simulink model "ADMIRE"  (R2021b)
settings: Solver=ode4  StartTime=0.0  StopTime=100  FixedStep=1e-2  RelTol=1e-3
undefined symbols (not defined in the file or in its folder): admireDB, Earth, WGS84
libraries: simulink_extras x112, simulink x27, aerolibutil x4, dspsigops x4, aerolibfltsims x3, sharedtransform x2, aerolibtransform2 x2, aerolibatmos2 x1, matrix_library x1, sharedutil x1, aerolibanimutils x1, vrlib x1
(part 2 of 15)

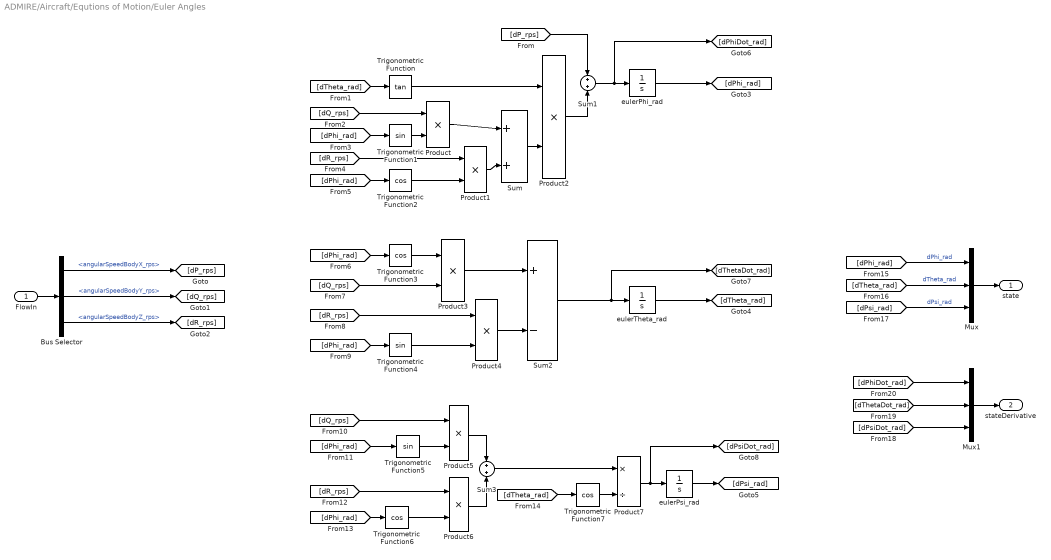
== system ADMIRE/Aircraft/Equtions of Motion/Euler Angles ==
  FlowIn : Inport
  Bus Selector : BusSelector  OutputSignals=EOM_Bus.angularSpeedBodyX_rps,EOM_Bus.angularSpeedBodyY_rps,EOM_Bus.angularSpeedBodyZ_rps
  Mux : Mux  Inputs=3
  Mux1 : Mux  Inputs=3
  Product{,1..6} (7 alike) : Product
  Product7 : Product  Inputs=*/
  Sum : Sum  Inputs=+|+
  Sum1 : Sum  Inputs=+|+
  Sum2 : Sum  Inputs=+-
  Sum3 : Sum  Inputs=+|+
  Trigonometric Function : Trigonometry  Operator=tan
  Trigonometric Function1 : Trigonometry
  Trigonometric Function{2..3,6..7} (4 alike) : Trigonometry  Operator=cos
  Trigonometric Function4 : Trigonometry
  Trigonometric Function5 : Trigonometry
  eulerPhi_rad : Integrator  WrapState=on  ContinuousStateAttributes='eulerPhi_rad'
  eulerPsi_rad : Integrator  WrapState=on  WrappedStateUpperValue=2*pi  WrappedStateLowerValue=0  ContinuousStateAttributes='eulerPsi_rad'
  eulerTheta_rad : Integrator  WrapState=on  WrappedStateUpperValue=pi/2  WrappedStateLowerValue=-pi/2  ContinuousStateAttributes='eulerTheta_rad'
  state : Outport
  stateDerivative : Outport  Port=2
  wires:
  Mux/1 -> state/1
  [dR_rps] -> Product1/1
  eulerPhi_rad/1 -> [dPhi_rad]
  [dTheta_rad] -> Mux/2  "dTheta_rad"
  Trigonometric Function7/1 -> Product7/2
  Sum1/1 -> [dPhiDot_rad], eulerPhi_rad/1
  [dPsi_rad] -> Mux/3  "dPsi_rad"
  [dPhi_rad] -> Mux/1  "dPhi_rad"
  Product4/1 -> Sum2/2
  Product6/1 -> Sum3/2
  Sum2/1 -> [dThetaDot_rad], eulerTheta_rad/1
  [dPhi_rad] -> Trigonometric Function1/1
  Product5/1 -> Sum3/1
  Trigonometric Function4/1 -> Product4/2
  [dPhi_rad] -> Trigonometric Function2/1
  Trigonometric Function6/1 -> Product6/2
  Product3/1 -> Sum2/1
  [dQ_rps] -> Product3/2
  [dPhi_rad] -> Trigonometric Function6/1
  Trigonometric Function5/1 -> Product5/2
  [dPhi_rad] -> Trigonometric Function5/1
  Product1/1 -> Sum/2
  [dR_rps] -> Product4/1
  Trigonometric Function2/1 -> Product1/2
  [dTheta_rad] -> Trigonometric Function/1
  Sum/1 -> Product2/2
  Trigonometric Function1/1 -> Product/2
  Trigonometric Function/1 -> Product2/1
  Product2/1 -> Sum1/2
  eulerTheta_rad/1 -> [dTheta_rad]
  Sum3/1 -> Product7/1
  [dTheta_rad] -> Trigonometric Function7/1
  [dQ_rps] -> Product/1
  [dR_rps] -> Product6/1
  [dP_rps] -> Sum1/1
  Product/1 -> Sum/1
  [dPhi_rad] -> Trigonometric Function3/1
  [dPhi_rad] -> Trigonometric Function4/1
  Product7/1 -> eulerPsi_rad/1, [dPsiDot_rad]
  Trigonometric Function3/1 -> Product3/1
  eulerPsi_rad/1 -> [dPsi_rad]
  [dQ_rps] -> Product5/1
  FlowIn/1 -> Bus Selector/1
  Bus Selector/3 -> [dR_rps]  "<angularSpeedBodyZ_rps>"
  Bus Selector/2 -> [dQ_rps]  "<angularSpeedBodyY_rps>"
  Bus Selector/1 -> [dP_rps]  "<angularSpeedBodyX_rps>"
  [dPhiDot_rad] -> Mux1/1
  [dThetaDot_rad] -> Mux1/2
  [dPsiDot_rad] -> Mux1/3
  Mux1/1 -> stateDerivative/1

== system ADMIRE/Aircraft/Equtions of Motion/Navigation ==
  FlowIn : Inport
  Bus Selector : BusSelector  OutputSignals=DCM_Bus.dcmBody2NED,EOM_Bus.speedBodyX_mps,EOM_Bus.speedBodyY_mps,EOM_Bus.speedBodyZ_mps
  Demux : Demux  Outputs=3
  Gain : Gain  Gain=-1
  Matrix Multiply : Product  Multiplication=Matrix(*)
  Mux : Mux  Inputs=3
  Mux1 : Mux  Inputs=3
  altitude_m : Integrator  ContinuousStateAttributes='altitude_m'
  positionEarthX_m : Integrator  ContinuousStateAttributes='positionEarthX_m'
  positionEarthY_m : Integrator  ContinuousStateAttributes='positionEarthY_m'
  state : Outport
  stateDerivative : Outport  Port=2
  wires:
  FlowIn/1 -> Bus Selector/1
  Bus Selector/2 -> Mux/1  "<speedBodyX_mps>"
  Bus Selector/3 -> Mux/2  "<speedBodyY_mps>"
  Bus Selector/4 -> Mux/3  "<speedBodyZ_mps>"
  Bus Selector/1 -> Matrix Multiply/1  "<dcmBody2NED>"
  Mux/1 -> Matrix Multiply/2
  Matrix Multiply/1 -> stateDerivative/1, Demux/1
  Demux/1 -> positionEarthX_m/1
  Demux/2 -> positionEarthY_m/1
  Demux/3 -> Gain/1
  positionEarthY_m/1 -> Mux1/2
  positionEarthX_m/1 -> Mux1/1
  altitude_m/1 -> Mux1/3
  Mux1/1 -> state/1
  Gain/1 -> altitude_m/1

== system ADMIRE/Aircraft/Equtions of Motion/Translational Speeds ==
  Flow : Inport
  Angle of Attack Equation : Subsystem
  Angle of Sideslip Equation : Subsystem
  ForcesWindAxes : Subsystem
  Mux : Mux  Inputs=6
  Selector : Selector  InputPortWidth=6  IndexOptions=Index vector (dialog)  Indices=[1 3 5]  OutputSizes=1
  Selector1 : Selector  InputPortWidth=6  IndexOptions=Index vector (dialog)  Indices=[2 4 6]  OutputSizes=1
  V Equation : Subsystem
  state : Outport
  stateDerivative : Outport  Port=2
  wires:
  V Equation/1(V) -> Mux/1  "V"
  Angle of Sideslip Equation/1(aos) -> Mux/5  "aos"
  Angle of Attack Equation/1(aoa) -> Mux/3  "aoa"
  Flow/1 -> Angle of Sideslip Equation/2(Flow), Angle of Attack Equation/2(Flow), V Equation/2(Flow), ForcesWindAxes/1(Flow)
  Mux/1 -> Selector1/1, Selector/1
  V Equation/2(VDot) -> Mux/2  "VDot"
  Angle of Attack Equation/2(aoaDot) -> Mux/4  "aoaDot"
  Angle of Sideslip Equation/2(aosDot) -> Mux/6  "aosDot"
  Selector/1 -> state/1
  Selector1/1 -> stateDerivative/1
  ForcesWindAxes/1(ForcesWindAxes) -> Angle of Attack Equation/1(ForcesWindAxes), Angle of Sideslip Equation/1(ForcesWindAxes), V Equation/1(ForcesWindAxes)

== system ADMIRE/Aircraft/Mass/Inertia ==
  Create 3x3 Matrix : sharedutil/Create 3x3 Matrix  aMode=aMode
      settings: SourceProductBaseCode=AE,PW,DR,MT,UV,VE
  Gain : Gain  Gain=-1
  Gain1 : Gain  Gain=-1
  Gain2 : Gain  Gain=-1
  "Ix " : Constant  Value=21000
  Ixy : Constant  Value=0
  "Ixz " : Constant  Value=2500
  "Iy " : Constant  Value=81000
  Iyz : Constant  Value=0
  "Iz " : Constant  Value=101000
  InertiaTensor : Outport
  inertiaIx_kgpm2 : Outport  Port=2
  inertiaIy_kgpm2 : Outport  Port=3
  inertiaIz_kgpm2 : Outport  Port=4
  inertiaIxy_kgpm2 : Outport  Port=5
  inertiaIxz_kgpm2 : Outport  Port=6
  inertiaIyz_kgpm2 : Outport  Port=7
  wires:
  "Ix "/1 -> Create 3x3 Matrix/1, [Ix]
  "Iz "/1 -> [Iz], Create 3x3 Matrix/9
  Gain2/1 -> Create 3x3 Matrix/6, Create 3x3 Matrix/8
  [Iy] -> inertiaIy_kgpm2/1  "inertiaIy_kgpm2"
  "Ixz "/1 -> [Ixz], Gain1/1
  Ixy/1 -> [Ixy], Gain/1
  Create 3x3 Matrix/1 -> InertiaTensor/1  "InertiaTensor"
  [Ix] -> inertiaIx_kgpm2/1  "inertiaIx_kgpm2"
  Gain/1 -> Create 3x3 Matrix/4, Create 3x3 Matrix/2
  [Iyz] -> inertiaIyz_kgpm2/1  "inertiaIyz_kgpm2"
  Gain1/1 -> Create 3x3 Matrix/7, Create 3x3 Matrix/3
  "Iy "/1 -> [Iy], Create 3x3 Matrix/5
  Iyz/1 -> [Iyz], Gain2/1
  [Ixz] -> inertiaIxz_kgpm2/1  "inertiaIxz_kgpm2"
  [Ixy] -> inertiaIxy_kgpm2/1  "inertiaIxy_kgpm2"
  [Iz] -> inertiaIz_kgpm2/1  "inertiaIz_kgpm2"

== system ADMIRE/InputSelection/LogitechExtremePro3D/Subsystem ==
  JoyInput : Inport
  TrimInput : Inport  Port=2
  Constant1 : Constant
  Gain : Gain  Gain=20
  Integrator : Integrator  InitialConditionSource=external
  Sample and Hold : dspsigops/Sample and Hold  trig=Either edge  initCond=0  latchinput=off
  Sum : Sum  Inputs=|+-
  Switch : Switch  Criteria=u2 > Threshold
  Out : Outport
  wires:
  Constant1/1 -> Sample and Hold/1
  Sample and Hold/1 -> Switch/2
  JoyInput/1 -> Sample and Hold/Trigger, Switch/1
  Switch/1 -> Sum/1
  TrimInput/1 -> Integrator/2, Switch/3
  Integrator/1 -> Out/1, Sum/2
  Sum/1 -> Gain/1
  Gain/1 -> Integrator/1

== system ADMIRE/InputSelection/LogitechExtremePro3D/Subsystem1 ==
  JoyInput : Inport
  TrimInput : Inport  Port=2
  Constant1 : Constant
  Gain : Gain  Gain=20
  Integrator : Integrator  InitialConditionSource=external
  Sample and Hold : dspsigops/Sample and Hold  trig=Either edge  initCond=0  latchinput=off
  Sum : Sum  Inputs=|+-
  Switch : Switch  Criteria=u2 > Threshold
  Out : Outport
  wires:
  Gain/1 -> Integrator/1
  Sum/1 -> Gain/1
  Integrator/1 -> Sum/2, Out/1
  TrimInput/1 -> Switch/3, Integrator/2
  Switch/1 -> Sum/1
  JoyInput/1 -> Switch/1, Sample and Hold/Trigger
  Sample and Hold/1 -> Switch/2
  Constant1/1 -> Sample and Hold/1

== system ADMIRE/InputSelection/LogitechExtremePro3D/Subsystem2 ==
  JoyInput : Inport
  TrimInput : Inport  Port=2
  Constant1 : Constant
  Gain : Gain  Gain=20
  Integrator : Integrator  InitialConditionSource=external
  Sample and Hold : dspsigops/Sample and Hold  trig=Either edge  initCond=0  latchinput=off
  Sum : Sum  Inputs=|+-
  Switch : Switch  Criteria=u2 > Threshold
  Out : Outport
  wires:
  Constant1/1 -> Sample and Hold/1
  Sample and Hold/1 -> Switch/2
  JoyInput/1 -> Sample and Hold/Trigger, Switch/1
  Switch/1 -> Sum/1
  TrimInput/1 -> Integrator/2, Switch/3
  Integrator/1 -> Out/1, Sum/2
  Sum/1 -> Gain/1
  Gain/1 -> Integrator/1

== system ADMIRE/InputSelection/LogitechExtremePro3D/Subsystem3 ==
  JoyInput : Inport
  TrimInput : Inport  Port=2
  Constant1 : Constant
  Gain : Gain  Gain=20
  Integrator : Integrator  InitialConditionSource=external
  Sample and Hold : dspsigops/Sample and Hold  trig=Either edge  initCond=0  latchinput=off
  Sum : Sum  Inputs=|+-
  Switch : Switch  Criteria=u2 > Threshold
  Out : Outport
  wires:
  Gain/1 -> Integrator/1
  Sum/1 -> Gain/1
  Integrator/1 -> Sum/2, Out/1
  TrimInput/1 -> Switch/3, Integrator/2
  Switch/1 -> Sum/1
  JoyInput/1 -> Switch/1, Sample and Hold/Trigger
  Sample and Hold/1 -> Switch/2
  Constant1/1 -> Sample and Hold/1

== system ADMIRE/Aircraft/Aerodynamics/CentripetalForceCoefficient/MachRegion1 ==
  note: Mach <= 0.4
  AeroIn_Bus : Inport
  Bus Creator : BusCreator  Inputs=3
  Ccbcai : Subsystem
  Ccbde : Subsystem
  Ccbdle : Subsystem
  Ccbdn : Subsystem
  Ccbeta : Subsystem
  Ccbetad : Subsystem
  Ccblg : Subsystem
  Ccdai : Subsystem
  Ccdaib : Subsystem
  Ccday : Subsystem
  Ccdayb : Subsystem
  Ccdna : Subsystem
  Ccdr : Subsystem
  Ccp : Subsystem
  Ccpbeta : Subsystem
  Ccr : Subsystem
  Ccrbeta : Subsystem
  Sum : Sum  Inputs=17
  eoeff1 : Subsystem
  cctot : Outport
  wires:
  Ccrbeta/1(Ccrbeta) -> Sum/17  "Ccrbeta"
  Ccr/1(Ccr) -> Sum/16  "Ccr"
  Ccpbeta/1(Ccpbeta) -> Sum/15  "Ccpbeta"
  Ccp/1(Ccp) -> Sum/14  "Ccp"
  Ccbetad/1(Ccbetad) -> Sum/13  "Ccbetad"
  Ccdna/1(Ccdna) -> Sum/12  "Ccdna"
  Ccdayb/1(Ccdayb) -> Sum/11  "Ccdayb"
  Ccday/1(Ccday) -> Sum/10  "Ccday"
  Ccdaib/1(Ccdaib) -> Sum/9  "Ccdaib"
  Ccdai/1(Ccdai) -> Sum/8  "Ccdai"
  Ccdr/1(Ccdr) -> Sum/7  "Ccdr"
  Ccbcai/1(Ccbcai) -> Sum/6  "Ccbcai"
  Ccbdle/1(Ccbdle) -> Sum/5  "Ccbdle"
  Ccbdn/1(Ccbdn) -> Sum/4  "Ccbdn"
  Ccbde/1(Ccbde) -> Sum/3  "Ccbde"
  Ccblg/1(Ccblg) -> Sum/2  "Ccblg"
  Ccbeta/1(Ccbeta) -> Sum/1  "Ccbeta"
  Bus Creator/1 -> Ccp/1(in_bus), Ccpbeta/1(in_bus), Ccr/1(in_bus), Ccrbeta/1(in_bus), Ccbetad/1(in_bus), Ccdna/1(in_bus), Ccdayb/1(in_bus), Ccday/1(in_bus), Ccdaib/1(in_bus), Ccdai/1(in_bus), Ccdr/1(in_bus), Ccbcai/1(in_bus), Ccbdle/1(in_bus), Ccbdn/1(in_bus), Ccbde/1(in_bus), Ccblg/1(in_bus), Ccbeta/1(in_bus)  "in_bus"
  eoeff1/2(eieff) -> Bus Creator/3  "eieff"
  AeroIn_Bus/1 -> eoeff1/1(AeroIn_Bus), Bus Creator/1
  eoeff1/1(eoeff) -> Bus Creator/2  "eoeff"
  Sum/1 -> cctot/1

== system ADMIRE/Aircraft/Aerodynamics/CentripetalForceCoefficient/MachRegion2 ==
  note: 0.4 < Mach < 0.5
  AeroIn_Bus : Inport
  Bus Creator : BusCreator  Inputs=3
  Ccbcai : Subsystem
  Ccbde : Subsystem
  Ccbdle : Subsystem
  Ccbdn : Subsystem
  Ccbeta : Subsystem
  Ccbetad : Subsystem
  Ccblg : Subsystem
  Ccdai : Subsystem
  Ccdaib : Subsystem
  Ccday : Subsystem
  Ccdayb : Subsystem
  Ccdna : Subsystem
  Ccdr : Subsystem
  Ccp : Subsystem
  Ccpbeta : Subsystem
  Ccr : Subsystem
  Ccrbeta : Subsystem
  Sum : Sum  Inputs=17
  eoeff1 : Subsystem
  cctot : Outport
  wires:
  Ccrbeta/1(Ccrbeta) -> Sum/17  "Ccrbeta"
  Ccr/1(Ccr) -> Sum/16  "Ccr"
  Ccpbeta/1(Ccpbeta) -> Sum/15  "Ccpbeta"
  Ccp/1(Ccp) -> Sum/14  "Ccp"
  Ccbetad/1(Ccbetad) -> Sum/13  "Ccbetad"
  Ccdna/1(Ccdna) -> Sum/12  "Ccdna"
  Ccdayb/1(Ccdayb) -> Sum/11  "Ccdayb"
  Ccday/1(Ccday) -> Sum/10  "Ccday"
  Ccdaib/1(Ccdaib) -> Sum/9  "Ccdaib"
  Ccdai/1(Ccdai) -> Sum/8  "Ccdai"
  Ccdr/1(Ccdr) -> Sum/7  "Ccdr"
  Ccbcai/1(Ccbcai) -> Sum/6  "Ccbcai"
  Ccbdle/1(Ccbdle) -> Sum/5  "Ccbdle"
  Ccbdn/1(Ccbdn) -> Sum/4  "Ccbdn"
  Ccbde/1(Ccbde) -> Sum/3  "Ccbde"
  Ccblg/1(Ccblg) -> Sum/2  "Ccblg"
  Ccbeta/1(Ccbeta) -> Sum/1  "Ccbeta"
  Bus Creator/1 -> Ccr/1(in_bus), Ccrbeta/1(in_bus), Ccpbeta/1(in_bus), Ccp/1(in_bus), Ccbetad/1(in_bus), Ccdna/1(in_bus), Ccdayb/1(in_bus), Ccday/1(in_bus), Ccdaib/1(in_bus), Ccdai/1(in_bus), Ccdr/1(in_bus), Ccbcai/1(in_bus), Ccbdle/1(in_bus), Ccbdn/1(in_bus), Ccbde/1(in_bus), Ccblg/1(in_bus), Ccbeta/1(in_bus)  "in_bus"
  eoeff1/1(eoeff) -> Bus Creator/2  "eoeff"
  eoeff1/2(eieff) -> Bus Creator/3  "eieff"
  AeroIn_Bus/1 -> eoeff1/1(AeroIn_Bus), Bus Creator/1
  Sum/1 -> cctot/1

== system ADMIRE/Aircraft/Aerodynamics/CentripetalForceCoefficient/MachRegion3 ==
  note: 0.5 <= Mach <= 1.4
  AeroIn_Bus : Inport
  Bus Creator : BusCreator  Inputs=3
  Ccbcai : Subsystem
  Ccbde : Subsystem
  Ccbdle : Subsystem
  Ccbdn : Subsystem
  Ccbeta : Subsystem
  Ccbetad : Subsystem
  Ccblg : Subsystem
  Ccdai : Subsystem
  Ccdaib : Subsystem
  Ccday : Subsystem
  Ccdayb : Subsystem
  Ccdna : Subsystem
  Ccdr : Subsystem
  Ccp1 : Subsystem
  Ccpbeta : Subsystem
  Ccr1 : Subsystem
  Ccrbeta : Subsystem
  Sum : Sum  Inputs=17
  eoeff1 : Subsystem
  cctot : Outport
  wires:
  Ccrbeta/1(Ccrbeta) -> Sum/17  "Ccrbeta"
  Ccr1/1(Ccr) -> Sum/16  "Ccr"
  Ccpbeta/1(Ccpbeta) -> Sum/15  "Ccpbeta"
  Ccp1/1(Ccp) -> Sum/14  "Ccp"
  Ccbetad/1(Ccbetad) -> Sum/13  "Ccbetad"
  Ccdna/1(Ccdna) -> Sum/12  "Ccdna"
  Ccdayb/1(Ccdayb) -> Sum/11  "Ccdayb"
  Ccday/1(Ccday) -> Sum/10  "Ccday"
  Ccdaib/1(Ccdaib) -> Sum/9  "Ccdaib"
  Ccdai/1(Ccdai) -> Sum/8  "Ccdai"
  Ccdr/1(Ccdr) -> Sum/7  "Ccdr"
  Ccbcai/1(Ccbcai) -> Sum/6  "Ccbcai"
  Ccbdle/1(Ccbdle) -> Sum/5  "Ccbdle"
  Ccbdn/1(Ccbdn) -> Sum/4  "Ccbdn"
  Ccbde/1(Ccbde) -> Sum/3  "Ccbde"
  Ccblg/1(Ccblg) -> Sum/2  "Ccblg"
  Ccbeta/1(Ccbeta) -> Sum/1  "Ccbeta"
  eoeff1/2(eieff) -> Bus Creator/3  "eieff"
  eoeff1/1(eoeff) -> Bus Creator/2  "eoeff"
  Bus Creator/1 -> Ccr1/1(in_bus), Ccp1/1(in_bus), Ccbetad/1(in_bus), Ccdna/1(in_bus), Ccday/1(in_bus), Ccdai/1(in_bus), Ccdr/1(in_bus), Ccbcai/1(in_bus), Ccbdle/1(in_bus), Ccbdn/1(in_bus), Ccbde/1(in_bus), Ccblg/1(in_bus), Ccbeta/1(in_bus)  "in_bus"
  AeroIn_Bus/1 -> eoeff1/1(AeroIn_Bus), Bus Creator/1
  Sum/1 -> cctot/1

== system ADMIRE/Aircraft/Aerodynamics/CentripetalForceCoefficient/MachRegion4 ==
  note: 1.4 < Mach
  AeroIn_Bus : Inport
  Bus Creator : BusCreator  Inputs=3
  Ccbcai : Subsystem
  Ccbde : Subsystem
  Ccbdle : Subsystem
  Ccbdn : Subsystem
  Ccbeta : Subsystem
  Ccbetad : Subsystem
  Ccblg : Subsystem
  Ccdai : Subsystem
  Ccdaib : Subsystem
  Ccday : Subsystem
  Ccdayb : Subsystem
  Ccdna : Subsystem
  Ccdr : Subsystem
  Ccp : Subsystem
  Ccpbeta : Subsystem
  Ccr : Subsystem
  Ccrbeta : Subsystem
  Sum : Sum  Inputs=17
  eoeff : Subsystem
  cttot : Outport
  wires:
  Ccrbeta/1(Ccrbeta) -> Sum/17  "Ccrbeta"
  Ccr/1(Ccr) -> Sum/16  "Ccr"
  Ccpbeta/1(Ccpbeta) -> Sum/15  "Ccpbeta"
  Ccp/1(Ccp) -> Sum/14  "Ccp"
  Ccbetad/1(Ccbetad) -> Sum/13  "Ccbetad"
  Ccdna/1(Ccdna) -> Sum/12  "Ccdna"
  Ccdayb/1(Ccdayb) -> Sum/11  "Ccdayb"
  Ccday/1(Ccday) -> Sum/10  "Ccday"
  Ccdaib/1(Ccdaib) -> Sum/9  "Ccdaib"
  Ccdai/1(Ccdai) -> Sum/8  "Ccdai"
  Ccblg/1(Ccblg) -> Sum/7  "Ccblg"
  Ccdr/1(Ccdr) -> Sum/6  "Ccdr"
  Ccbcai/1(Ccbcai) -> Sum/5  "Ccbcai"
  Ccbdle/1(Ccbdle) -> Sum/4  "Ccbdle"
  Ccbdn/1(Ccbdn) -> Sum/3  "Ccbdn"
  Ccbde/1(Ccbde) -> Sum/2  "Ccbde"
  Ccbeta/1(Ccbeta) -> Sum/1  "Ccbeta"
  AeroIn_Bus/1 -> eoeff/1(AeroIn_Bus), Bus Creator/1
  Bus Creator/1 -> Ccbde/1(in_bus), Ccbdn/1(in_bus), Ccbdle/1(in_bus), Ccbcai/1(in_bus), Ccdr/1(in_bus), Ccr/1(in_bus), Ccp/1(in_bus), Ccbetad/1(in_bus), Ccdna/1(in_bus), Ccday/1(in_bus), Ccdai/1(in_bus), Ccblg/1(in_bus), Ccbeta/1(in_bus)  "in_bus"
  eoeff/2(eieff) -> Bus Creator/3  "eieff"
  eoeff/1(eoeff) -> Bus Creator/2  "eoeff"
  Sum/1 -> cttot/1

== system ADMIRE/Aircraft/Aerodynamics/CentripetalForceCoefficient/Subsystem ==
  mach_nd : Inport
  CctotMR1 : Inport  Port=2
  CctotMR2 : Inport  Port=3
  CctotMR3 : Inport  Port=4
  CctotMR4 : Inport  Port=5
  AND : Logic  IconShape=distinctive  AllPortsSameDT=off  OutDataTypeStr=boolean
  AND1 : Logic  IconShape=distinctive  AllPortsSameDT=off  OutDataTypeStr=boolean
  Compare To Constant1 : simulink/Logic and Bit Operations/Compare To Constant  relop=<=  const=0.4  OutDataTypeStr=boolean
  Compare To Constant2 : simulink/Logic and Bit Operations/Compare To Constant  relop=>  const=0.4  OutDataTypeStr=boolean
  Compare To Constant3 : simulink/Logic and Bit Operations/Compare To Constant  relop=<  const=0.5  OutDataTypeStr=boolean
  Compare To Constant4 : simulink/Logic and Bit Operations/Compare To Constant  relop=<=  const=1.4  OutDataTypeStr=boolean
  Compare To Constant5 : simulink/Logic and Bit Operations/Compare To Constant  relop=>=  const=0.5  OutDataTypeStr=boolean
  Switch : Switch  Criteria=u2 ~= 0
  Switch1 : Switch  Criteria=u2 ~= 0
  Switch2 : Switch  Criteria=u2 ~= 0
  Cctot : Outport
  wires:
  Switch/1 -> Cctot/1
  Compare To Constant5/1 -> AND1/1
  Compare To Constant4/1 -> AND1/2
  AND1/1 -> Switch2/2
  CctotMR4/1 -> Switch2/3
  CctotMR3/1 -> Switch2/1
  CctotMR1/1 -> Switch/1
  Switch2/1 -> Switch1/3
  CctotMR2/1 -> Switch1/1
  Switch1/1 -> Switch/3
  AND/1 -> Switch1/2
  Compare To Constant3/1 -> AND/2
  Compare To Constant2/1 -> AND/1
  Compare To Constant1/1 -> Switch/2
  mach_nd/1 -> Compare To Constant1/1, Compare To Constant3/1, Compare To Constant4/1, Compare To Constant5/1, Compare To Constant2/1

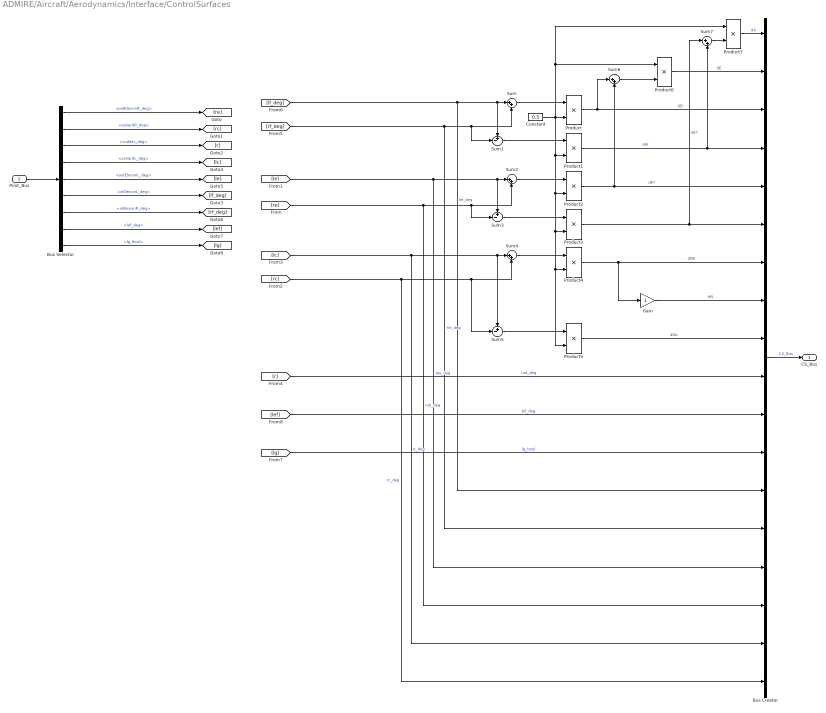
== system ADMIRE/Aircraft/Aerodynamics/Interface/ControlSurfaces ==
  Pilot_Bus : Inport
  Bus Creator : BusCreator  Inputs=18
  Bus Selector : BusSelector  OutputSignals=CS_Bus.outElevonR_deg,CS_Bus.canardR_deg,CS_Bus.rudder_deg,CS_Bus.canardL_deg,CS_Bus.outElevonL_deg,CS_Bus.inElevonL_deg,CS_Bus.inElevonR_deg,CS_Bus.lef_deg,CS_Bus.lg_bool
  Constant : Constant  Value=0.5
  Gain : Gain
  Product{,1..7} (8 alike) : Product
  Sum{,2,4,6..7} (5 alike) : Sum  Inputs=|++
  Sum1 : Sum  Inputs=+-|
  Sum3 : Sum  Inputs=+-|
  Sum5 : Sum  Inputs=+-|
  CS_Bus : Outport
  wires:
  Product/1 -> Sum6/1, Bus Creator/3  "dEI"
  [lf_deg] -> Bus Creator/13, Sum1/1, Sum/1  "lie_deg"
  Product1/1 -> Sum7/2, Bus Creator/4  "dAI"
  Product2/1 -> Sum6/2, Bus Creator/5  "dEY"
  Product3/1 -> Bus Creator/6, Sum7/1  "dAY"
  Product5/1 -> Bus Creator/9  "dNA"
  Product4/1 -> Gain/1, Bus Creator/7  "dNE"
  Gain/1 -> Bus Creator/8  "dN"
  Constant/1 -> Product7/1, Product6/1, Product5/2, Product4/2, Product3/2, Product2/2, Product1/2, Product/2
  Sum6/1 -> Product6/2
  Product6/1 -> Bus Creator/2  "dE"
  Bus Creator/1 -> CS_Bus/1  "CS_Bus"
  [lg] -> Bus Creator/12  "lg_bool"
  Sum/1 -> Product/1
  Sum2/1 -> Product2/1
  Sum1/1 -> Product1/1
  Sum3/1 -> Product3/1
  Sum4/1 -> Product4/1
  Sum5/1 -> Product5/1
  Sum7/1 -> Product7/2
  Product7/1 -> Bus Creator/1  "dA"
  [rf_deg] -> Bus Creator/14, Sum1/2, Sum/2  "rie_deg"
  [le] -> Sum2/1, Sum3/1, Bus Creator/15  "loe_deg"
  [re] -> Sum3/2, Sum2/2, Bus Creator/16  "roe_deg"
  [lc] -> Sum5/1, Sum4/1, Bus Creator/17  "lc_deg"
  [rc] -> Bus Creator/18, Sum5/2, Sum4/2  "rc_deg"
  [r] -> Bus Creator/10  "rud_deg"
  [lef] -> Bus Creator/11  "lef_deg"
  Pilot_Bus/1 -> Bus Selector/1
  Bus Selector/1 -> [re]  "<outElevonR_deg>"
  Bus Selector/2 -> [rc]  "<canardR_deg>"
  Bus Selector/3 -> [r]  "<rudder_deg>"
  Bus Selector/4 -> [lc]  "<canardL_deg>"
  Bus Selector/5 -> [le]  "<outElevonL_deg>"
  Bus Selector/7 -> [rf_deg]  "<inElevonR_deg>"
  Bus Selector/6 -> [lf_deg]  "<inElevonL_deg>"
  Bus Selector/8 -> [lef]  "<lef_deg>"
  Bus Selector/9 -> [lg]  "<lg_bool>"

== system ADMIRE/Aircraft/Aerodynamics/Interface/Subsystem ==
  In1 : Inport
  Bus Selector : BusSelector  OutputSignals=AC_Bus.referenceChord_m,EOM_Bus.speedWindX_mps,AC_Bus.referenceSpan_m,EOM_Bus.angleOfAttackDot_rps2,EOM_Bus.angleOfSideslipDot_rps2,EOM_Bus.angularSpeedBodyX_rps,EOM_Bus.angularSpeedBodyY_rps,EOM_Bus.angularSpeedBodyZ_rps
  Constant : Constant  Value=2
  Constant1 : Constant  Value=0.1
  Max : MinMax  Function=max  Inputs=2
  Product : Product  Inputs=*/
  Product1 : Product  Inputs=*/
  Product2 : Product  Inputs=/*
  Product3 : Product  Inputs=/*
  Product{4..8} (5 alike) : Product
  angleOfAttackRate_nd : Outport
  anglefOfSideslipRate_nd : Outport  Port=2
  rollRate_nd : Outport  Port=3
  pitchRate_nd : Outport  Port=4
  yawRate_nd : Outport  Port=5
  wires:
  In1/1 -> Bus Selector/1
  Constant/1 -> Product3/1, Product2/1
  Product1/1 -> Product3/2
  Bus Selector/2 -> Max/2  "<speedWindX_mps>"
  Bus Selector/1 -> Product/1  "<referenceChord_m>"
  Product/1 -> Product2/2
  Bus Selector/3 -> Product1/1  "<referenceSpan_m>"
  Product7/1 -> pitchRate_nd/1  "pitchRate_nd"
  Product5/1 -> anglefOfSideslipRate_nd/1  "anglefOfSideslipRate_nd"
  Product3/1 -> Product5/2, Product6/2, Product8/2
  Product6/1 -> rollRate_nd/1  "rollRate_nd"
  Product2/1 -> Product4/2, Product7/2
  Product8/1 -> yawRate_nd/1  "yawRate_nd"
  Product4/1 -> angleOfAttackRate_nd/1  "angleOfAttackRate_nd"
  Bus Selector/4 -> Product4/1  "<angleOfAttackDot_rps2>"
  Bus Selector/5 -> Product5/1  "<angleOfSideslipDot_rps2>"
  Bus Selector/6 -> Product6/1  "<angularSpeedBodyX_rps>"
  Bus Selector/8 -> Product8/1  "<angularSpeedBodyZ_rps>"
  Bus Selector/7 -> Product7/1  "<angularSpeedBodyY_rps>"
  Max/1 -> Product1/2, Product/2
  Constant1/1 -> Max/1

== system ADMIRE/Aircraft/Aerodynamics/NormalForceCoefficient/MachRegion1 ==
  note: Mach <= 0.4
  Misc_Bus : Inport
  Bus Creator : BusCreator  Inputs=3
  Cnalfa : Subsystem
  Cnalfad : Subsystem
  Cnbasic : Subsystem
  Cnbeta : Subsystem
  Cncai : Subsystem
  Cndedn : Subsystem
  Cndei : Subsystem
  Cndey : Subsystem
  Cndle : Subsystem
  Cndn : Subsystem
  Cnhigh : Subsystem
  Cnlg : Subsystem
  Cnnz : Subsystem
  Cnq : Subsystem
  Cnqd : Subsystem
  Sum : Sum  Inputs=15
  eoeff : Subsystem
  Cntot : Outport
  wires:
  Sum/1 -> Cntot/1
  Cnhigh/1(Cnhigh) -> Sum/15  "Cnhigh"
  Cnqd/1(Cnqd) -> Sum/14  "Cnqd"
  Cnnz/1(Cnnz) -> Sum/13  "Cnnz"
  Cnq/1(Cnq) -> Sum/12  "Cnq"
  Cnalfad/1(Cnalfad) -> Sum/11  "Cnalfad"
  Cnlg/1(Cnlg) -> Sum/10  "Cnlg"
  Cnbeta/1(Cnbeta) -> Sum/9  "Cnbeta"
  Cncai/1(Cncai) -> Sum/8  "Cncai"
  Cndle/1(Cndle) -> Sum/7  "Cndle"
  Cndn/1(Cndn) -> Sum/6  "Cndn"
  Cndedn/1(Cndedn) -> Sum/5  "Cndedn"
  Cndey/1(Cndey) -> Sum/4  "Cndey"
  Cndei/1(Cndei) -> Sum/3  "Cndei"
  Cnalfa/1(Cnalfa) -> Sum/2  "Cnalfa"
  Cnbasic/1(Cnbasic) -> Sum/1  "Cnbasic"
  Bus Creator/1 -> Cnbasic/1(in_bus), Cnalfa/1(in_bus), Cndei/1(in_bus), Cndey/1(in_bus), Cndedn/1(in_bus), Cndn/1(in_bus), Cndle/1(in_bus), Cncai/1(in_bus), Cnbeta/1(in_bus), Cnlg/1(in_bus), Cnalfad/1(in_bus), Cnq/1(in_bus), Cnnz/1(in_bus), Cnqd/1(in_bus), Cnhigh/1(in_bus)  "in_bus"
  eoeff/1(eoeff) -> Bus Creator/2  "eoeff"
  Misc_Bus/1 -> eoeff/1(AeroIn_Bus), Bus Creator/1
  eoeff/2(eieff) -> Bus Creator/3  "eieff"

== system ADMIRE/Aircraft/Aerodynamics/NormalForceCoefficient/MachRegion2 ==
  note: 0.4 < Mach < 0.5
  Misc_Bus : Inport
  Bus Creator : BusCreator  Inputs=3
  Cnalfa : Subsystem
  Cnalfad : Subsystem
  Cnbasic : Subsystem
  Cnbeta : Subsystem
  Cncai : Subsystem
  Cndedn : Subsystem
  Cndei : Subsystem
  Cndey : Subsystem
  Cndle : Subsystem
  Cndn : Subsystem
  Cnhigh : Subsystem
  Cnlg : Subsystem
  Cnnz : Subsystem
  Cnq : Subsystem
  Cnqd : Subsystem
  Sum : Sum  Inputs=15
  eoeff : Subsystem
  Cntot : Outport
  wires:
  Sum/1 -> Cntot/1
  eoeff/2(eieff) -> Bus Creator/3  "eieff"
  Misc_Bus/1 -> Bus Creator/1, eoeff/1(AeroIn_Bus)
  eoeff/1(eoeff) -> Bus Creator/2  "eoeff"
  Bus Creator/1 -> Cnqd/1(in_bus), Cnnz/1(in_bus), Cnq/1(in_bus), Cnalfad/1(in_bus), Cnlg/1(in_bus), Cnbeta/1(in_bus), Cncai/1(in_bus), Cndle/1(in_bus), Cndn/1(in_bus), Cndedn/1(in_bus), Cndey/1(in_bus), Cndei/1(in_bus), Cnalfa/1(in_bus), Cnbasic/1(in_bus)  "in_bus"
  Cnbasic/1(Cnbasic) -> Sum/1  "Cnbasic"
  Cnalfa/1(Cnalfa) -> Sum/2  "Cnalfa"
  Cndei/1(Cndei) -> Sum/3  "Cndei"
  Cndey/1(Cndey) -> Sum/4  "Cndey"
  Cndedn/1(Cndedn) -> Sum/5  "Cndedn"
  Cndn/1(Cndn) -> Sum/6  "Cndn"
  Cndle/1(Cndle) -> Sum/7  "Cndle"
  Cncai/1(Cncai) -> Sum/8  "Cncai"
  Cnbeta/1(Cnbeta) -> Sum/9  "Cnbeta"
  Cnlg/1(Cnlg) -> Sum/10  "Cnlg"
  Cnalfad/1(Cnalfad) -> Sum/11  "Cnalfad"
  Cnq/1(Cnq) -> Sum/12  "Cnq"
  Cnnz/1(Cnnz) -> Sum/13  "Cnnz"
  Cnqd/1(Cnqd) -> Sum/14  "Cnqd"
  Cnhigh/1(Cnhigh) -> Sum/15  "Cnhigh"

== system ADMIRE/Aircraft/Aerodynamics/NormalForceCoefficient/MachRegion3 ==
  note: 0.5 <= Mach
  Misc_Bus : Inport
  Bus Creator : BusCreator  Inputs=3
  Cnalfa : Subsystem
  Cnalfad : Subsystem
  Cnbasic : Subsystem
  Cnbeta : Subsystem
  Cncai : Subsystem
  Cndedn : Subsystem
  Cndei : Subsystem
  Cndey : Subsystem
  Cndle : Subsystem
  Cndn : Subsystem
  Cnhigh : Subsystem
  Cnlg : Subsystem
  Cnnz : Subsystem
  Cnq : Subsystem
  Cnqd : Subsystem
  Sum : Sum  Inputs=15
  eoeff : Subsystem
  Cntot : Outport
  wires:
  Sum/1 -> Cntot/1
  eoeff/2(eieff) -> Bus Creator/3  "eieff"
  Misc_Bus/1 -> Bus Creator/1, eoeff/1(AeroIn_Bus)
  eoeff/1(eoeff) -> Bus Creator/2  "eoeff"
  Bus Creator/1 -> Cnqd/1(in_bus), Cnnz/1(in_bus), Cnq/1(in_bus), Cnalfad/1(in_bus), Cnlg/1(in_bus), Cncai/1(in_bus), Cndle/1(in_bus), Cndn/1(in_bus), Cndey/1(in_bus), Cndei/1(in_bus), Cnalfa/1(in_bus), Cnbasic/1(in_bus)  "in_bus"
  Cnbasic/1(Cnbasic) -> Sum/1  "Cnbasic"
  Cnalfa/1(Cnalfa) -> Sum/2  "Cnalfa"
  Cndei/1(Cndei) -> Sum/3  "Cndei"
  Cndey/1(Cndey) -> Sum/4  "Cndey"
  Cndedn/1(Cndedn) -> Sum/5  "Cndedn"
  Cndn/1(Cndn) -> Sum/6  "Cndn"
  Cndle/1(Cndle) -> Sum/7  "Cndle"
  Cncai/1(Cncai) -> Sum/8  "Cncai"
  Cnbeta/1(Cnbeta) -> Sum/9  "Cnbeta"
  Cnlg/1(Cnlg) -> Sum/10  "Cnlg"
  Cnalfad/1(Cnalfad) -> Sum/11  "Cnalfad"
  Cnq/1(Cnq) -> Sum/12  "Cnq"
  Cnnz/1(Cnnz) -> Sum/13  "Cnnz"
  Cnqd/1(Cnqd) -> Sum/14  "Cnqd"
  Cnhigh/1(Cnhigh) -> Sum/15  "Cnhigh"

== system ADMIRE/Aircraft/Aerodynamics/NormalForceCoefficient/Subsystem ==
  mach_nd : Inport
  CntotMR1 : Inport  Port=2
  CntotMR2 : Inport  Port=3
  CntotMR3 : Inport  Port=4
  AND : Logic  IconShape=distinctive  AllPortsSameDT=off  OutDataTypeStr=boolean
  Compare To Constant1 : simulink/Logic and Bit Operations/Compare To Constant  relop=<=  const=0.4  OutDataTypeStr=boolean
  Compare To Constant2 : simulink/Logic and Bit Operations/Compare To Constant  relop=>  const=0.4  OutDataTypeStr=boolean
  Compare To Constant3 : simulink/Logic and Bit Operations/Compare To Constant  relop=<  const=0.5  OutDataTypeStr=boolean
  Switch : Switch  Criteria=u2 ~= 0
  Switch1 : Switch  Criteria=u2 ~= 0
  Cntot : Outport
  wires:
  Switch/1 -> Cntot/1
  CntotMR3/1 -> Switch1/3
  CntotMR2/1 -> Switch1/1
  Switch1/1 -> Switch/3
  CntotMR1/1 -> Switch/1
  AND/1 -> Switch1/2
  Compare To Constant3/1 -> AND/2
  Compare To Constant2/1 -> AND/1
  Compare To Constant1/1 -> Switch/2
  mach_nd/1 -> Compare To Constant1/1, Compare To Constant3/1, Compare To Constant2/1

== system ADMIRE/Aircraft/Aerodynamics/PitchMomentCoefficient/MachRegion1 ==
  note: Mach <= 0.4
  Misc_Bus : Inport
  Bus Creator : BusCreator  Inputs=3
  Cpmalfa : Subsystem
  Cpmalfad : Subsystem
  Cpmbasic : Subsystem
  Cpmbeta : Subsystem
  Cpmcai : Subsystem
  Cpmda : Subsystem
  Cpmdedn : Subsystem
  Cpmdei : Subsystem
  Cpmdey : Subsystem
  Cpmdle : Subsystem
  Cpmdn : Subsystem
  Cpmhigh : Subsystem
  Cpmlg : Subsystem
  Cpmnz : Subsystem
  Cpmq : Subsystem
  Cpmqd : Subsystem
  Sum : Sum  Inputs=16
  eoeff : Subsystem
  Cpmtot : Outport
  wires:
  Cpmhigh/1(Cpmhigh) -> Sum/16  "Cpmhigh"
  Cpmqd/1(Cpmqd) -> Sum/15  "Cpmqd"
  Cpmnz/1(Cpmnz) -> Sum/14  "Cpmnz"
  Cpmq/1(Cpmq) -> Sum/13  "Cpmq"
  Cpmalfad/1(Cpmalfad) -> Sum/12  "Cpmalfad"
  Cpmda/1(Cpmda) -> Sum/11  "Cpmda"
  Cpmbasic/1(Cpmbasic) -> Sum/1  "Cpmbasic"
  Cpmbeta/1(Cpmbeta) -> Sum/10  "Cpmbeta"
  Cpmalfa/1(Cpmalfa) -> Sum/2  "Cpmalfa"
  Cpmcai/1(Cpmcai) -> Sum/9  "Cpmcai"
  Cpmdei/1(Cpmdei) -> Sum/3  "Cpmdei"
  Cpmlg/1(Cpmlg) -> Sum/8  "Cpmlg"
  Cpmdey/1(Cpmdey) -> Sum/4  "Cpmdey"
  Cpmdle/1(Cpmdle) -> Sum/7  "Cpmdle"
  Cpmdedn/1(Cpmdedn) -> Sum/5  "Cpmdedn"
  Cpmdn/1(Cpmdn) -> Sum/6  "Cpmdn"
  Bus Creator/1 -> Cpmbasic/1(in_bus), Cpmnz/1(in_bus), Cpmqd/1(in_bus), Cpmhigh/1(in_bus), Cpmq/1(in_bus), Cpmalfad/1(in_bus), Cpmda/1(in_bus), Cpmbeta/1(in_bus), Cpmcai/1(in_bus), Cpmlg/1(in_bus), Cpmdle/1(in_bus), Cpmdn/1(in_bus), Cpmdedn/1(in_bus), Cpmdey/1(in_bus), Cpmdei/1(in_bus), Cpmalfa/1(in_bus)  "in_bus"
  eoeff/1(eoeff) -> Bus Creator/2  "eoeff"
  eoeff/2(eieff) -> Bus Creator/3  "eieff"
  Misc_Bus/1 -> eoeff/1(AeroIn_Bus), Bus Creator/1
  Sum/1 -> Cpmtot/1

== system ADMIRE/Aircraft/Aerodynamics/PitchMomentCoefficient/MachRegion2 ==
  note: 0.4 < Mach < 0.5
  Misc_Bus : Inport
  Bus Creator : BusCreator  Inputs=5
  Cpmalfa : Subsystem
  Cpmalfad : Subsystem
  Cpmbasic : Subsystem
  Cpmbeta : Subsystem
  Cpmcai : Subsystem
  Cpmda : Subsystem
  Cpmdedn : Subsystem
  Cpmdei : Subsystem
  Cpmdey : Subsystem
  Cpmdle : Subsystem
  Cpmdn : Subsystem
  Cpmhigh : Subsystem
  Cpmlg : Subsystem
  Cpmnz : Subsystem
  Cpmq : Subsystem
  Cpmqd : Subsystem
  Sum : Sum  Inputs=16
  eoeff : Subsystem
  Cpmtot : Outport
  wires:
  eoeff/3(eoefflow) -> Bus Creator/4  "eoefflow"
  eoeff/4(eiefflow) -> Bus Creator/5  "eiefflow"
  Sum/1 -> Cpmtot/1
  Misc_Bus/1 -> Bus Creator/1, eoeff/1(AeroIn_Bus)
  eoeff/2(eieff) -> Bus Creator/3  "eieff"
  eoeff/1(eoeff) -> Bus Creator/2  "eoeff"
  Bus Creator/1 -> Cpmalfa/1(in_bus), Cpmdei/1(in_bus), Cpmdedn/1(in_bus), Cpmdn/1(in_bus), Cpmdle/1(in_bus), Cpmlg/1(in_bus), Cpmcai/1(in_bus), Cpmbeta/1(in_bus), Cpmda/1(in_bus), Cpmalfad/1(in_bus), Cpmq/1(in_bus), Cpmqd/1(in_bus), Cpmnz/1(in_bus), Cpmdey/1(in_bus), Cpmbasic/1(in_bus)  "in_bus"
  Cpmdn/1(Cpmdn) -> Sum/6  "Cpmdn"
  Cpmdedn/1(Cpmdedn) -> Sum/5  "Cpmdedn"
  Cpmdle/1(Cpmdle) -> Sum/7  "Cpmdle"
  Cpmdey/1(Cpmdey) -> Sum/4  "Cpmdey"
  Cpmlg/1(Cpmlg) -> Sum/8  "Cpmlg"
  Cpmdei/1(Cpmdei) -> Sum/3  "Cpmdei"
  Cpmcai/1(Cpmcai) -> Sum/9  "Cpmcai"
  Cpmalfa/1(Cpmalfa) -> Sum/2  "Cpmalfa"
  Cpmbeta/1(Cpmbeta) -> Sum/10  "Cpmbeta"
  Cpmbasic/1(Cpmbasic) -> Sum/1  "Cpmbasic"
  Cpmda/1(Cpmda) -> Sum/11  "Cpmda"
  Cpmalfad/1(Cpmalfad) -> Sum/12  "Cpmalfad"
  Cpmq/1(Cpmq) -> Sum/13  "Cpmq"
  Cpmnz/1(Cpmnz) -> Sum/14  "Cpmnz"
  Cpmqd/1(Cpmqd) -> Sum/15  "Cpmqd"
  Cpmhigh/1(Cpmhigh) -> Sum/16  "Cpmhigh"

== system ADMIRE/Aircraft/Aerodynamics/PitchMomentCoefficient/MachRegion3 ==
  note: 0.5 <= Mach
  Misc_Bus : Inport
  Bus Creator : BusCreator  Inputs=3
  Cpmalfa : Subsystem
  Cpmalfad : Subsystem
  Cpmbasic : Subsystem
  Cpmbeta : Subsystem
  Cpmcai : Subsystem
  Cpmda : Subsystem
  Cpmdedn : Subsystem
  Cpmdei : Subsystem
  Cpmdey : Subsystem
  Cpmdle : Subsystem
  Cpmdn : Subsystem
  Cpmhigh : Subsystem
  Cpmlg : Subsystem
  Cpmnz : Subsystem
  Cpmq : Subsystem
  Cpmqd : Subsystem
  Sum : Sum  Inputs=16
  eoeff : Subsystem
  Cpmtot : Outport
  wires:
  Sum/1 -> Cpmtot/1
  Misc_Bus/1 -> Bus Creator/1, eoeff/1(AeroIn_Bus)
  eoeff/2(eieff) -> Bus Creator/3  "eieff"
  eoeff/1(eoeff) -> Bus Creator/2  "eoeff"
  Bus Creator/1 -> Cpmalfa/1(in_bus), Cpmdei/1(in_bus), Cpmdn/1(in_bus), Cpmdle/1(in_bus), Cpmlg/1(in_bus), Cpmcai/1(in_bus), Cpmalfad/1(in_bus), Cpmq/1(in_bus), Cpmqd/1(in_bus), Cpmnz/1(in_bus), Cpmdey/1(in_bus), Cpmbasic/1(in_bus)  "in_bus"
  Cpmdn/1(Cpmdn) -> Sum/6  "Cpmdn"
  Cpmdedn/1(Cpmdedn) -> Sum/5  "Cpmdedn"
  Cpmdle/1(Cpmdle) -> Sum/7  "Cpmdle"
  Cpmdey/1(Cpmdey) -> Sum/4  "Cpmdey"
  Cpmlg/1(Cpmlg) -> Sum/8  "Cpmlg"
  Cpmdei/1(Cpmdei) -> Sum/3  "Cpmdei"
  Cpmcai/1(Cpmcai) -> Sum/9  "Cpmcai"
  Cpmalfa/1(Cpmalfa) -> Sum/2  "Cpmalfa"
  Cpmbeta/1(Cpmbeta) -> Sum/10  "Cpmbeta"
  Cpmbasic/1(Cpmbasic) -> Sum/1  "Cpmbasic"
  Cpmda/1(Cpmda) -> Sum/11  "Cpmda"
  Cpmalfad/1(Cpmalfad) -> Sum/12  "Cpmalfad"
  Cpmq/1(Cpmq) -> Sum/13  "Cpmq"
  Cpmnz/1(Cpmnz) -> Sum/14  "Cpmnz"
  Cpmqd/1(Cpmqd) -> Sum/15  "Cpmqd"
  Cpmhigh/1(Cpmhigh) -> Sum/16  "Cpmhigh"

== system ADMIRE/Aircraft/Aerodynamics/PitchMomentCoefficient/Subsystem ==
  mach_nd : Inport
  CpmtotMR1 : Inport  Port=2
  CpmtotMR2 : Inport  Port=3
  CpmtotMR3 : Inport  Port=4
  AND : Logic  IconShape=distinctive  AllPortsSameDT=off  OutDataTypeStr=boolean
  Compare To Constant1 : simulink/Logic and Bit Operations/Compare To Constant  relop=<=  const=0.4  OutDataTypeStr=boolean
  Compare To Constant2 : simulink/Logic and Bit Operations/Compare To Constant  relop=>  const=0.4  OutDataTypeStr=boolean
  Compare To Constant3 : simulink/Logic and Bit Operations/Compare To Constant  relop=<  const=0.5  OutDataTypeStr=boolean
  Switch : Switch  Criteria=u2 ~= 0
  Switch1 : Switch  Criteria=u2 ~= 0
  Cpmtot : Outport
  wires:
  Switch/1 -> Cpmtot/1
  CpmtotMR3/1 -> Switch1/3
  CpmtotMR2/1 -> Switch1/1
  Switch1/1 -> Switch/3
  CpmtotMR1/1 -> Switch/1
  AND/1 -> Switch1/2
  Compare To Constant3/1 -> AND/2
  Compare To Constant2/1 -> AND/1
  Compare To Constant1/1 -> Switch/2
  mach_nd/1 -> Compare To Constant1/1, Compare To Constant3/1, Compare To Constant2/1

== system ADMIRE/Aircraft/Aerodynamics/RollMomentCoefficient/MachRegion1 ==
  note: Mach <= 0.4
  AeroIn_Bus : Inport
  Bus Creator : BusCreator  Inputs=3
  Crmbasic : Subsystem
  Crmbde : Subsystem
  Crmbdle : Subsystem
  Crmbdn : Subsystem
  Crmbeta : Subsystem
  Crmbetad : Subsystem
  Crmblg : Subsystem
  Crmdai : Subsystem
  Crmdaib : Subsystem
  Crmday : Subsystem
  Crmdayb : Subsystem
  Crmdna : Subsystem
  Crmdr : Subsystem
  Crmp : Subsystem
  Crmpbeta : Subsystem
  Crmr : Subsystem
  Crmrbeta : Subsystem
  Crmrde : Subsystem
  Sum : Sum  Inputs=18
  eoeff1 : Subsystem
  crmtot : Outport
  wires:
  Crmrde/1(Crmrbeta) -> Sum/18  "Crmrde"
  Crmrbeta/1(Crmrbeta) -> Sum/17  "Crmrbeta"
  Crmr/1(Crmr) -> Sum/16  "Crmr"
  Crmpbeta/1(Crmpbeta) -> Sum/15  "Crmpbeta"
  Crmp/1(Crmp) -> Sum/14  "Crmp"
  Crmbetad/1(Crmbetad) -> Sum/13  "Crmbetad"
  Crmdna/1(Crmdna) -> Sum/12  "Crmdna"
  Crmdayb/1(Crmdayb) -> Sum/11  "Crmdayb"
  Crmday/1(Crmday) -> Sum/10  "Crmday"
  Crmdaib/1(Crmdaib) -> Sum/9  "Crmdaib"
  Crmdai/1(Crmdai) -> Sum/8  "Crmdai"
  Crmdr/1(Crmdr) -> Sum/7  "Crmdr"
  Crmblg/1(Crmblg) -> Sum/6  "Crmblg"
  Crmbdle/1(Crmbdle) -> Sum/5  "Crmbdle"
  Crmbdn/1(Crmbdn) -> Sum/4  "Crmbdn"
  Crmbde/1(Crmbde) -> Sum/3  "Crmbde"
  Crmbeta/1(Crmbeta) -> Sum/2  "Crmbeta"
  Crmbasic/1(Crmbasic) -> Sum/1  "Crmbasic"
  eoeff1/1(eoeff) -> Bus Creator/2  "eoeff"
  Bus Creator/1 -> Crmr/1(in_bus), Crmrbeta/1(in_bus), Crmrde/1(in_bus), Crmpbeta/1(in_bus), Crmp/1(in_bus), Crmbetad/1(in_bus), Crmdna/1(in_bus), Crmdayb/1(in_bus), Crmday/1(in_bus), Crmdaib/1(in_bus), Crmdai/1(in_bus), Crmdr/1(in_bus), Crmblg/1(in_bus), Crmbdle/1(in_bus), Crmbdn/1(in_bus), Crmbde/1(in_bus), Crmbeta/1(in_bus), Crmbasic/1(in_bus)  "in_bus"
  AeroIn_Bus/1 -> eoeff1/1(AeroIn_Bus), Bus Creator/1
  eoeff1/2(eieff) -> Bus Creator/3  "eieff"
  Sum/1 -> crmtot/1

== system ADMIRE/Aircraft/Aerodynamics/RollMomentCoefficient/MachRegion2 ==
  note: 0.4 < Mach < 0.5
  AeroIn_Bus : Inport
  Bus Creator : BusCreator  Inputs=3
  Crmbasic : Subsystem
  Crmbde : Subsystem
  Crmbdle : Subsystem
  Crmbdn : Subsystem
  Crmbeta : Subsystem
  Crmbetad : Subsystem
  Crmblg : Subsystem
  Crmdai : Subsystem
  Crmdaib : Subsystem
  Crmday : Subsystem
  Crmdayb : Subsystem
  Crmdna : Subsystem
  Crmdr : Subsystem
  Crmp : Subsystem
  Crmpbeta : Subsystem
  Crmr : Subsystem
  Crmrbeta : Subsystem
  Crmrde : Subsystem
  Sum : Sum  Inputs=18
  eoeff1 : Subsystem
  crmtot : Outport
  wires:
  Crmpbeta/1(Crmpbeta) -> Sum/15  "Crmpbeta"
  Crmdaib/1(Crmdaib) -> Sum/9  "Crmdaib"
  Crmdai/1(Crmdai) -> Sum/8  "Crmdai"
  Crmbasic/1(Crmbasic) -> Sum/1  "Crmbasic"
  Crmrbeta/1(Crmrbeta) -> Sum/17  "Crmrbeta"
  Crmr/1(Crmr) -> Sum/16  "Crmr"
  Crmdna/1(Crmdna) -> Sum/12  "Crmdna"
  Sum/1 -> crmtot/1
  Crmbetad/1(Crmbetad) -> Sum/13  "Crmbetad"
  Crmp/1(Crmp) -> Sum/14  "Crmp"
  AeroIn_Bus/1 -> eoeff1/1(AeroIn_Bus), Bus Creator/1
  Crmdayb/1(Crmdayb) -> Sum/11  "Crmdayb"
  eoeff1/2(eieff) -> Bus Creator/3  "eieff"
  Crmdr/1(Crmdr) -> Sum/7  "Crmdr"
  Crmbdn/1(Crmbdn) -> Sum/4  "Crmbdn"
  Crmbde/1(Crmbde) -> Sum/3  "Crmbde"
  eoeff1/1(eoeff) -> Bus Creator/2  "eoeff"
  Bus Creator/1 -> Crmr/1(in_bus), Crmrbeta/1(in_bus), Crmrde/1(in_bus), Crmpbeta/1(in_bus), Crmp/1(in_bus), Crmbetad/1(in_bus), Crmdna/1(in_bus), Crmdayb/1(in_bus), Crmday/1(in_bus), Crmdaib/1(in_bus), Crmdai/1(in_bus), Crmdr/1(in_bus), Crmblg/1(in_bus), Crmbdle/1(in_bus), Crmbdn/1(in_bus), Crmbde/1(in_bus), Crmbeta/1(in_bus), Crmbasic/1(in_bus)  "in_bus"
  Crmbdle/1(Crmbdle) -> Sum/5  "Crmbdle"
  Crmday/1(Crmday) -> Sum/10  "Crmday"
  Crmblg/1(Crmblg) -> Sum/6  "Crmblg"
  Crmbeta/1(Crmbeta) -> Sum/2  "Crmbeta"
  Crmrde/1(Crmrde) -> Sum/18  "Crmrde"

== system ADMIRE/Aircraft/Aerodynamics/RollMomentCoefficient/MachRegion3 ==
  note: 0.5 <= Mach <= 1.4
  AeroIn_Bus : Inport
  Bus Creator : BusCreator  Inputs=3
  Crmbasic : Subsystem
  Crmbde : Subsystem
  Crmbdle : Subsystem
  Crmbdn : Subsystem
  Crmbeta : Subsystem
  Crmbetad : Subsystem
  Crmblg : Subsystem
  Crmdai : Subsystem
  Crmdaib : Subsystem
  Crmday : Subsystem
  Crmdayb : Subsystem
  Crmdna : Subsystem
  Crmdr : Subsystem
  Crmp : Subsystem
  Crmpbeta : Subsystem
  Crmr : Subsystem
  Crmrbeta : Subsystem
  Crmrde : Subsystem
  Sum : Sum  Inputs=18
  eoeff1 : Subsystem
  crmtot : Outport
  wires:
  Sum/1 -> crmtot/1
  Crmrde/1(Crmrde) -> Sum/18  "Crmrde"
  Crmrbeta/1(Crmrbeta) -> Sum/17  "Crmrbeta"
  Crmr/1(Crmr) -> Sum/16  "Crmr"
  Crmpbeta/1(Crmpbeta) -> Sum/15  "Crmpbeta"
  Crmp/1(Crmp) -> Sum/14  "Crmp"
  Crmbetad/1(Crmbetad) -> Sum/13  "Crmbetad"
  Crmdna/1(Crmdna) -> Sum/12  "Crmdna"
  Crmdayb/1(Crmdayb) -> Sum/11  "Crmdayb"
  Crmday/1(Crmday) -> Sum/10  "Crmday"
  Crmdaib/1(Crmdaib) -> Sum/9  "Crmdaib"
  Crmdai/1(Crmdai) -> Sum/8  "Crmdai"
  Crmdr/1(Crmdr) -> Sum/7  "Crmdr"
  Crmblg/1(Crmblg) -> Sum/6  "Crmblg"
  Crmbdle/1(Crmbdle) -> Sum/5  "Crmbdle"
  Crmbdn/1(Crmbdn) -> Sum/4  "Crmbdn"
  Crmbde/1(Crmbde) -> Sum/3  "Crmbde"
  Crmbeta/1(Crmbeta) -> Sum/2  "Crmbeta"
  Crmbasic/1(Crmbasic) -> Sum/1  "Crmbasic"
  eoeff1/2(eieff) -> Bus Creator/3  "eieff"
  eoeff1/1(eoeff) -> Bus Creator/2  "eoeff"
  Bus Creator/1 -> Crmr/1(in_bus), Crmrde/1(in_bus), Crmp/1(in_bus), Crmbetad/1(in_bus), Crmdna/1(in_bus), Crmday/1(in_bus), Crmdai/1(in_bus), Crmdr/1(in_bus), Crmblg/1(in_bus), Crmbdle/1(in_bus), Crmbdn/1(in_bus), Crmbde/1(in_bus), Crmbeta/1(in_bus)  "in_bus"
  AeroIn_Bus/1 -> eoeff1/1(AeroIn_Bus), Bus Creator/1

== system ADMIRE/Aircraft/Aerodynamics/RollMomentCoefficient/MachRegion4 ==
  note: 1.4 < Mach
  AeroIn_Bus : Inport
  Bus Creator : BusCreator  Inputs=3
  Crmbasic : Subsystem
  Crmbde : Subsystem
  Crmbdle : Subsystem
  Crmbdn : Subsystem
  Crmbeta : Subsystem
  Crmbetad : Subsystem
  Crmblg : Subsystem
  Crmdai : Subsystem
  Crmdaib : Subsystem
  Crmday : Subsystem
  Crmdayb : Subsystem
  Crmdna : Subsystem
  Crmdr : Subsystem
  Crmp : Subsystem
  Crmpbeta : Subsystem
  Crmr : Subsystem
  Crmrbeta : Subsystem
  Crmrde : Subsystem
  Sum : Sum  Inputs=18
  eoeff1 : Subsystem
  crmtot : Outport
  wires:
  Crmrde/1(Crmrde) -> Sum/18  "Crmrde"
  Crmrbeta/1(Crmrbeta) -> Sum/17  "Crmrbeta"
  Crmr/1(Crmr) -> Sum/16  "Crmr"
  Crmpbeta/1(Crmpbeta) -> Sum/15  "Crmpbeta"
  Crmp/1(Crmp) -> Sum/14  "Crmp"
  Crmbetad/1(Crmbetad) -> Sum/13  "Crmbetad"
  Crmdna/1(Crmdna) -> Sum/12  "Crmdna"
  Crmdayb/1(Crmdayb) -> Sum/11  "Crmdayb"
  Crmday/1(Crmday) -> Sum/10  "Crmday"
  Crmdaib/1(Crmdaib) -> Sum/9  "Crmdaib"
  Crmdai/1(Crmdai) -> Sum/8  "Crmdai"
  Crmdr/1(Crmdr) -> Sum/7  "Crmdr"
  Crmblg/1(Crmblg) -> Sum/6  "Crmblg"
  Crmbdle/1(Crmbdle) -> Sum/5  "Crmbdle"
  Crmbdn/1(Crmbdn) -> Sum/4  "Crmbdn"
  Crmbde/1(Crmbde) -> Sum/3  "Crmbde"
  Crmbeta/1(Crmbeta) -> Sum/2  "Crmbeta"
  Crmbasic/1(Crmbasic) -> Sum/1  "Crmbasic"
  eoeff1/1(eoeff) -> Bus Creator/2  "eoeff"
  AeroIn_Bus/1 -> eoeff1/1(AeroIn_Bus), Bus Creator/1
  Bus Creator/1 -> Crmr/1(in_bus), Crmrde/1(in_bus), Crmp/1(in_bus), Crmbetad/1(in_bus), Crmdna/1(in_bus), Crmday/1(in_bus), Crmdai/1(in_bus), Crmdr/1(in_bus), Crmblg/1(in_bus), Crmbdle/1(in_bus), Crmbdn/1(in_bus), Crmbde/1(in_bus), Crmbeta/1(in_bus)  "in_bus"
  eoeff1/2(eieff) -> Bus Creator/3  "eieff"
  Sum/1 -> crmtot/1

== system ADMIRE/Aircraft/Aerodynamics/RollMomentCoefficient/Subsystem ==
  mach_nd : Inport
  CrmtotMR1 : Inport  Port=2
  CrmtotMR2 : Inport  Port=3
  CrmtotMR3 : Inport  Port=4
  CrmtotMR4 : Inport  Port=5
  AND : Logic  IconShape=distinctive  AllPortsSameDT=off  OutDataTypeStr=boolean
  AND1 : Logic  IconShape=distinctive  AllPortsSameDT=off  OutDataTypeStr=boolean
  Compare To Constant1 : simulink/Logic and Bit Operations/Compare To Constant  relop=<=  const=0.4  OutDataTypeStr=boolean
  Compare To Constant2 : simulink/Logic and Bit Operations/Compare To Constant  relop=>  const=0.4  OutDataTypeStr=boolean
  Compare To Constant3 : simulink/Logic and Bit Operations/Compare To Constant  relop=<  const=0.5  OutDataTypeStr=boolean
  Compare To Constant4 : simulink/Logic and Bit Operations/Compare To Constant  relop=<=  const=1.4  OutDataTypeStr=boolean
  Compare To Constant5 : simulink/Logic and Bit Operations/Compare To Constant  relop=>=  const=0.5  OutDataTypeStr=boolean
  Switch : Switch  Criteria=u2 ~= 0
  Switch1 : Switch  Criteria=u2 ~= 0
  Switch2 : Switch  Criteria=u2 ~= 0
  Crmtot : Outport
  wires:
  Compare To Constant5/1 -> AND1/1
  Compare To Constant4/1 -> AND1/2
  AND1/1 -> Switch2/2
  CrmtotMR4/1 -> Switch2/3
  CrmtotMR3/1 -> Switch2/1
  Switch/1 -> Crmtot/1
  Switch2/1 -> Switch1/3
  CrmtotMR2/1 -> Switch1/1
  Switch1/1 -> Switch/3
  CrmtotMR1/1 -> Switch/1
  AND/1 -> Switch1/2
  Compare To Constant3/1 -> AND/2
  Compare To Constant2/1 -> AND/1
  Compare To Constant1/1 -> Switch/2
  mach_nd/1 -> Compare To Constant1/1, Compare To Constant3/1, Compare To Constant4/1, Compare To Constant5/1, Compare To Constant2/1

== system ADMIRE/Aircraft/Aerodynamics/TangentialForceCoefficient/MachRegion1 ==
  note: Mach <= 0.4
  AeroIn_Bus : Inport
  Bus Creator : BusCreator  Inputs=3
  Ctalfa : Subsystem
  Ctbasic : Subsystem
  Ctbeta : Subsystem
  Ctda : Subsystem
  Ctdedn : Subsystem
  Ctdei : Subsystem
  Ctdey : Subsystem
  Ctdle : Subsystem
  Ctdn : Subsystem
  Ctdr : Subsystem
  Cthigh : Subsystem
  Ctlg : Subsystem
  Sum : Sum  Inputs=12
  eoeff : Subsystem
  cttotMR1 : Outport
  wires:
  Ctdedn/1(Ctdedn) -> Sum/5  "Ctdedn"
  Ctdey/1(Ctdey) -> Sum/4  "Ctdey"
  Ctdei/1(Ctdei) -> Sum/3  "Ctdei"
  Ctalfa/1(Ctalfa) -> Sum/2  "Ctalfa"
  Ctbasic/1(Ctbasic) -> Sum/1  "Ctbasic"
  Cthigh/1(Cthigh) -> Sum/12  "Cthigh"
  Ctdr/1(Ctdr) -> Sum/11  "Ctdr"
  Ctda/1(Ctda) -> Sum/10  "Ctda"
  Ctbeta/1(Ctbeta) -> Sum/9  "Ctbeta"
  Ctlg/1(Ctlg) -> Sum/8  "Ctlg"
  Ctdle/1(Ctdle) -> Sum/7  "Ctdle"
  Ctdn/1(Ctdn) -> Sum/6  "Ctdn"
  Bus Creator/1 -> Ctbasic/1(in_bus), Ctalfa/1(in_bus), Ctdei/1(in_bus), Ctdey/1(in_bus), Ctdedn/1(in_bus), Ctdn/1(in_bus), Ctdle/1(in_bus), Ctlg/1(in_bus), Ctbeta/1(in_bus), Ctda/1(in_bus), Ctdr/1(in_bus), Cthigh/1(in_bus)  "in_bus"
  eoeff/2(eieff) -> Bus Creator/3  "eieff"
  eoeff/1(eoeff) -> Bus Creator/2  "eoeff"
  AeroIn_Bus/1 -> Bus Creator/1, eoeff/1(AeroIn_Bus)
  Sum/1 -> cttotMR1/1

== system ADMIRE/Aircraft/Aerodynamics/TangentialForceCoefficient/MachRegion2 ==
  note: 0.4 < Mach < 0.5
  AeroIn_Bus : Inport
  Bus Creator : BusCreator  Inputs=5
  Ctalfa : Subsystem
  Ctbasic : Subsystem
  Ctbeta : Subsystem
  Ctda : Subsystem
  Ctdedn : Subsystem
  Ctdei : Subsystem
  Ctdey : Subsystem
  Ctdle : Subsystem
  Ctdn : Subsystem
  Ctdr : Subsystem
  Cthigh : Subsystem
  Ctlg : Subsystem
  Sum : Sum  Inputs=12
  eoeff : Subsystem
  cttotMR2 : Outport
  wires:
  Cthigh/1(Cthigh) -> Sum/12  "Cthigh"
  Ctdr/1(Ctdr) -> Sum/11  "Ctdr"
  Ctda/1(Ctda) -> Sum/10  "Ctda"
  Ctbeta/1(Ctbeta) -> Sum/9  "Ctbeta"
  Ctlg/1(Ctlg) -> Sum/8  "Ctlg"
  Ctdle/1(Ctdle) -> Sum/7  "Ctdle"
  Ctdn/1(Ctdn) -> Sum/6  "Ctdn"
  eoeff/4(eieffhigh) -> Bus Creator/5  "eieffhigh"
  eoeff/3(eoeffhigh) -> Bus Creator/4  "eoeffhigh"
  Sum/1 -> cttotMR2/1
  AeroIn_Bus/1 -> Bus Creator/1
  eoeff/1(eoefflow) -> Bus Creator/2  "eoefflow"
  eoeff/2(eiefflow) -> Bus Creator/3  "eiefflow"
  Bus Creator/1 -> Ctdr/1(in_bus), Ctda/1(in_bus), Ctbeta/1(in_bus), Ctlg/1(in_bus), Ctdle/1(in_bus), Ctdn/1(in_bus), Ctdedn/1(in_bus), Ctdey/1(in_bus), Ctdei/1(in_bus), Ctalfa/1(in_bus), Ctbasic/1(in_bus)  "in_bus"
  Ctdei/1(Ctdei) -> Sum/3  "Ctdei"
  Ctalfa/1(Ctalfa) -> Sum/2  "Ctalfa"
  Ctdey/1(Ctdey) -> Sum/4  "Ctdey"
  Ctbasic/1(Ctbasic) -> Sum/1  "Ctbasic"
  Ctdedn/1(Ctdedn) -> Sum/5  "Ctdedn"

== system ADMIRE/Aircraft/Aerodynamics/TangentialForceCoefficient/MachRegion3 ==
  note: 0.5 < Mach
  AeroIn_Bus : Inport
  Bus Creator : BusCreator  Inputs=3
  Ctalfa : Subsystem
  Ctbasic : Subsystem
  Ctbeta : Subsystem
  Ctda : Subsystem
  Ctdedn : Subsystem
  Ctdei : Subsystem
  Ctdey : Subsystem
  Ctdle : Subsystem
  Ctdn : Subsystem
  Ctdr : Subsystem
  Cthigh : Subsystem
  Ctlg : Subsystem
  Sum : Sum  Inputs=12
  eoeff : Subsystem
  cttotMR3 : Outport
  wires:
  eoeff/2(eieff) -> Bus Creator/3  "eieff"
  eoeff/1(eoeff) -> Bus Creator/2  "eoeff"
  Cthigh/1(Cthigh) -> Sum/12  "Cthigh"
  Ctdr/1(Ctdr) -> Sum/11  "Ctdr"
  Ctda/1(Ctda) -> Sum/10  "Ctda"
  Ctbeta/1(Ctbeta) -> Sum/9  "Ctbeta"
  Ctlg/1(Ctlg) -> Sum/8  "Ctlg"
  Ctdle/1(Ctdle) -> Sum/7  "Ctdle"
  Ctdn/1(Ctdn) -> Sum/6  "Ctdn"
  Ctdedn/1(Ctdedn) -> Sum/5  "Ctdedn"
  Ctbasic/1(Ctbasic) -> Sum/1  "Ctbasic"
  Ctdey/1(Ctdey) -> Sum/4  "Ctdey"
  Ctalfa/1(Ctalfa) -> Sum/2  "Ctalfa"
  Ctdei/1(Ctdei) -> Sum/3  "Ctdei"
  Bus Creator/1 -> Ctbasic/1(in_bus), Ctalfa/1(in_bus), Ctdei/1(in_bus), Ctdn/1(in_bus), Ctdle/1(in_bus), Ctlg/1(in_bus), Ctda/1(in_bus), Ctdr/1(in_bus), Ctdey/1(in_bus)  "in_bus"
  AeroIn_Bus/1 -> eoeff/1(AeroIn_Bus), Bus Creator/1
  Sum/1 -> cttotMR3/1

== system ADMIRE/Aircraft/Aerodynamics/TangentialForceCoefficient/Subsystem ==
  mach_nd : Inport
  cttotMR1 : Inport  Port=2
  cttotMR2 : Inport  Port=3
  cttotMR3 : Inport  Port=4
  AND : Logic  IconShape=distinctive  AllPortsSameDT=off  OutDataTypeStr=boolean
  Compare To Constant1 : simulink/Logic and Bit Operations/Compare To Constant  relop=<=  const=0.4  OutDataTypeStr=boolean
  Compare To Constant2 : simulink/Logic and Bit Operations/Compare To Constant  relop=>  const=0.4  OutDataTypeStr=boolean
  Compare To Constant3 : simulink/Logic and Bit Operations/Compare To Constant  relop=<  const=0.5  OutDataTypeStr=boolean
  Switch : Switch  Criteria=u2 ~= 0
  Switch1 : Switch  Criteria=u2 ~= 0
  Out1 : Outport
  wires:
  Switch/1 -> Out1/1
  cttotMR3/1 -> Switch1/3
  cttotMR2/1 -> Switch1/1
  Switch1/1 -> Switch/3
  cttotMR1/1 -> Switch/1
  AND/1 -> Switch1/2
  Compare To Constant3/1 -> AND/2
  Compare To Constant2/1 -> AND/1
  Compare To Constant1/1 -> Switch/2
  mach_nd/1 -> Compare To Constant1/1, Compare To Constant3/1, Compare To Constant2/1

== system ADMIRE/Aircraft/Aerodynamics/YawMomentCoefficient/MachRegion1 ==
  note: Mach <= 0.4
  AeroIn_Bus : Inport
  Bus Creator : BusCreator  Inputs=3
  Cymbasic : Subsystem
  Cymbcai : Subsystem
  Cymbde : Subsystem
  Cymbdle : Subsystem
  Cymbdn : Subsystem
  Cymbeta : Subsystem
  Cymbetad : Subsystem
  Cymblg : Subsystem
  Cymdai : Subsystem
  Cymdaib : Subsystem
  Cymday : Subsystem
  Cymdayb : Subsystem
  Cymdna : Subsystem
  Cymdr : Subsystem
  Cymp : Subsystem
  Cympbeta : Subsystem
  Cymr : Subsystem
  Cymrbeta : Subsystem
  Sum : Sum  Inputs=18
  eoeff : Subsystem
  Cymtot : Outport
  wires:
  Cymbasic/1(Cymbasic) -> Sum/1  "Cymbasic"
  Cymbdn/1(Cymbdn) -> Sum/4  "Cymbdn"
  Cymbeta/1(Cymbeta) -> Sum/2  "Cymbeta"
  Cymbetad/1(Cymbetad) -> Sum/14  "Cymbetad"
  Cymday/1(Cymday) -> Sum/11  "Cymday"
  Cymp/1(Cymp) -> Sum/15  "Cymp"
  Cymdna/1(Cymdna) -> Sum/13  "Cymdna"
  eoeff/1(eoeff) -> Bus Creator/2  "eoeff"
  Cymr/1(Cymr) -> Sum/17  "Cymr"
  AeroIn_Bus/1 -> eoeff/1(AeroIn_Bus), Bus Creator/1
  Cymbde/1(Cymbde) -> Sum/3  "Cymbde"
  Cymbcai/1(Cymbcai) -> Sum/6  "Cymbcai"
  Cymblg/1(Cymblg) -> Sum/7  "Cymblg"
  Cymdaib/1(Cymdaib) -> Sum/10  "Cymdaib"
  Cymdai/1(Cymdai) -> Sum/9  "Cymdai"
  Cymdr/1(Cymdr) -> Sum/8  "Cymdr"
  Cymrbeta/1(Cymrbeta) -> Sum/18  "Cymrbeta"
  Bus Creator/1 -> Cympbeta/1(in_bus), Cymr/1(in_bus), Cymrbeta/1(in_bus), Cymp/1(in_bus), Cymbetad/1(in_bus), Cymdna/1(in_bus), Cymdayb/1(in_bus), Cymday/1(in_bus), Cymdaib/1(in_bus), Cymdai/1(in_bus), Cymdr/1(in_bus), Cymblg/1(in_bus), Cymbcai/1(in_bus), Cymbdle/1(in_bus), Cymbdn/1(in_bus), Cymbde/1(in_bus), Cymbeta/1(in_bus), Cymbasic/1(in_bus)  "in_bus"
  Cymdayb/1(Cymdayb) -> Sum/12  "Cymdayb"
  Cympbeta/1(Cympbeta) -> Sum/16  "Cympbeta"
  Cymbdle/1(Cymbdle) -> Sum/5  "Cymbdle"
  eoeff/2(eieff) -> Bus Creator/3  "eieff"
  Sum/1 -> Cymtot/1
